simulink model "wlan_agc"  (Simulink 7.8)
settings: Solver=VariableStepDiscrete  SolverMode=SingleTasking  StartTime=0.0  StopTime=1e4  RelTol=1e-3
PostLoadFcn:
  | wlan_agc_init
InitFcn:
  | wlan_agc_init
StartFcn:
  | wlan_agc_init
undefined symbols (not defined in the file): gcbh, PHY_CONFIG_PKT_DET_CORR_THRESH, PHY_CONFIG_PKT_DET_ENERGY_THRESH, PHY_CONFIG_PKT_DET_MIN_DURR, xlBlockLoadCallback, xlGetNormalizedPeriod
libraries: xbsIndex_r4 x991, xbsEDKLib_r4 x1, simulink x1
(part 4 of 7)

== system wlan_agc/DCO Correction/DCO Corr1 ==
  IQ Valid : Inport
  I : Inport  Port=2
  Q : Inport  Port=3
  Accumulator : xbsIndex_r4/Accumulator  operation=Add  n_bits=17  overflow=Flag as error  scale=1  rst=on  infoeditControl=reset for floating point data type must be asserted for a minimum of 2 cycles  hasbypass=off  en=on  latency=0  dbl_ovrd=off  msb_inp=100  msb=100  lsb=-100  use_behavioral_HDL=on  implementation=Fabric  block_type=accum
      settings: block_version=VER_STRING_GOES_HERE
  Accumulator1 : xbsIndex_r4/Accumulator  operation=Add  n_bits=17  overflow=Flag as error  scale=1  rst=on  infoeditControl=reset for floating point data type must be asserted for a minimum of 2 cycles  hasbypass=off  en=on  latency=0  dbl_ovrd=off  msb_inp=100  msb=100  lsb=-100  use_behavioral_HDL=on  implementation=Fabric  block_type=accum
      settings: block_version=VER_STRING_GOES_HERE
  AddSub : xbsIndex_r4/AddSub  mode=Subtraction  use_carryin=off  use_carryout=off  en=off  latency=1  precision=User Defined  arith_type="Signed  (2's comp)"  n_bits=16  bin_pt=15  quantization=Truncate  overflow=Wrap  dbl_ovrd=off  use_behavioral_HDL=off  hw_selection=Fabric  pipelined=off  block_type=addsub
  AddSub1 : xbsIndex_r4/AddSub  mode=Subtraction  use_carryin=off  use_carryout=off  en=off  latency=1  precision=User Defined  arith_type="Signed  (2's comp)"  n_bits=16  bin_pt=15  quantization=Truncate  overflow=Wrap  dbl_ovrd=off  use_behavioral_HDL=off  hw_selection=Fabric  pipelined=off  block_type=addsub
  Constant : xbsIndex_r4/Constant  const=31  gui_display_data_type=Fixed-point  arith_type=Unsigned  n_bits=5  bin_pt=0  preci_type=Single  exp_width=8  frac_width=24  explicit_period=off  period=1  equ=P=C  opselect=C  inp2=PCIN>>17  opr=+  inp1=P  carry=CIN  dbl_ovrd=off  block_type=constant
  Counter : xbsIndex_r4/Counter  cnt_type=Free Running  cnt_to=Inf  operation=Up  start_count=0  cnt_by_val=1  arith_type=Unsigned  n_bits=5  bin_pt=0  load_pin=off  rst=on  en=on  explicit_period=off  period=1  dbl_ovrd=off  use_behavioral_HDL=off  implementation=Fabric  block_type=counter
  DCO Est : Scope  NumInputPorts=7
      settings: TimeRange=10000  YMin=-0.4~-0.4~0~0~-0.02~-0.4~-0.4  YMax=0.4~0.4~1~0.03~0.009999999999999999~0.4~0.4
  Delay : xbsIndex_r4/Delay  rst=off  infoeditControl=Selection of Reset will increase slice count due to use of real FFs and instead of SRLs  en=off  latency=1  dbl_ovrd=off  reg_retiming=off  block_type=delay
  Logical : xbsIndex_r4/Logical  logical_function=AND  inputs=2  en=off  latency=0  precision=Full  arith_type=Unsigned  n_bits=16  bin_pt=0  align_bp=on  dbl_ovrd=off  block_type=logical
  Logical1 : xbsIndex_r4/Logical  logical_function=OR  inputs=2  en=off  latency=0  precision=Full  arith_type=Unsigned  n_bits=16  bin_pt=0  align_bp=on  dbl_ovrd=off  block_type=logical
  Logical2 : xbsIndex_r4/Logical  logical_function=AND  inputs=2  en=off  latency=0  precision=Full  arith_type=Unsigned  n_bits=16  bin_pt=0  align_bp=on  dbl_ovrd=off  block_type=logical
  Relational : xbsIndex_r4/Relational  mode=a=b  en=off  latency=0  dbl_ovrd=off  block_type=relational
  S-R Latch : Subsystem
  Scale : xbsIndex_r4/Scale  scale_factor=-5  dbl_ovrd=off  block_type=scale
  Scale1 : xbsIndex_r4/Scale  scale_factor=-5  dbl_ovrd=off  block_type=scale
  done{1..7} (7 alike) : xbsIndex_r4/Gateway Out  inherit_from_input=off  hdl_port=off  timing_constraint=None  locs_specified=off  LOCs={}  UseAsDAC=off  DACChannel='1'  block_type=gatewayout
      settings: infoedit="Gateway out block.  Converts Xilinx fixed point inputs into ouputs of type Simulink integer, double, or fixed point.<P><P>Hardware notes:  In hardware these blocks become top level output ports or are discarded, depending on how they are configured."  xl_area=[0 0 0 0 1 0 0]  block_version=VER_STRING_GOES_HERE
  Valid : Outport
  " I" : Outport  Port=2
  " Q" : Outport  Port=3
  wires:
  done7/1 -> DCO Est/7
  done1/1 -> DCO Est/6
  done3/1 -> DCO Est/4
  done5/1 -> DCO Est/3
  done6/1 -> DCO Est/5
  done2/1 -> DCO Est/2
  done4/1 -> DCO Est/1
  Scale1/1 -> done6/1, AddSub1/2
  Scale/1 -> done3/1, AddSub/2
  Logical2/1 -> Logical1/2
  Relational/1 -> Logical2/2
  Delay/1 -> Valid/1
  AddSub1/1 -> done7/1, " Q"/1
  AddSub/1 -> done1/1, " I"/1
  Logical1/1 -> Counter/1, S-R Latch/2(R)
  [AGC_RESET] -> Logical1/1
  Accumulator1/1 -> Scale1/1
  Accumulator/1 -> Scale/1
  IQ Valid/1 -> Logical2/1, Logical/1, Delay/1
  S-R Latch/1(Q) -> Logical/2
  Counter/1 -> Relational/1
  Constant/1 -> Relational/2
  Logical/1 -> done5/1, Accumulator/3, Accumulator1/3, Counter/2
  [AGC_CTRL_Start_DCO] -> S-R Latch/1(S)
  [AGC_RESET] -> Accumulator/2, Accumulator1/2
  Q/1 -> done2/1, AddSub1/1, Accumulator1/1
  I/1 -> done4/1, AddSub/1, Accumulator/1

== system wlan_agc/DCO Correction/DCO Corr2 ==
  IQ Valid : Inport
  I : Inport  Port=2
  Q : Inport  Port=3
  Accumulator : xbsIndex_r4/Accumulator  operation=Add  n_bits=17  overflow=Flag as error  scale=1  rst=on  infoeditControl=reset for floating point data type must be asserted for a minimum of 2 cycles  hasbypass=off  en=on  latency=0  dbl_ovrd=off  msb_inp=100  msb=100  lsb=-100  use_behavioral_HDL=on  implementation=Fabric  block_type=accum
      settings: block_version=VER_STRING_GOES_HERE
  Accumulator1 : xbsIndex_r4/Accumulator  operation=Add  n_bits=17  overflow=Flag as error  scale=1  rst=on  infoeditControl=reset for floating point data type must be asserted for a minimum of 2 cycles  hasbypass=off  en=on  latency=0  dbl_ovrd=off  msb_inp=100  msb=100  lsb=-100  use_behavioral_HDL=on  implementation=Fabric  block_type=accum
      settings: block_version=VER_STRING_GOES_HERE
  AddSub : xbsIndex_r4/AddSub  mode=Subtraction  use_carryin=off  use_carryout=off  en=off  latency=1  precision=User Defined  arith_type="Signed  (2's comp)"  n_bits=16  bin_pt=15  quantization=Truncate  overflow=Wrap  dbl_ovrd=off  use_behavioral_HDL=off  hw_selection=Fabric  pipelined=off  block_type=addsub
  AddSub1 : xbsIndex_r4/AddSub  mode=Subtraction  use_carryin=off  use_carryout=off  en=off  latency=1  precision=User Defined  arith_type="Signed  (2's comp)"  n_bits=16  bin_pt=15  quantization=Truncate  overflow=Wrap  dbl_ovrd=off  use_behavioral_HDL=off  hw_selection=Fabric  pipelined=off  block_type=addsub
  Constant : xbsIndex_r4/Constant  const=31  gui_display_data_type=Fixed-point  arith_type=Unsigned  n_bits=5  bin_pt=0  preci_type=Single  exp_width=8  frac_width=24  explicit_period=off  period=1  equ=P=C  opselect=C  inp2=PCIN>>17  opr=+  inp1=P  carry=CIN  dbl_ovrd=off  block_type=constant
  Counter : xbsIndex_r4/Counter  cnt_type=Free Running  cnt_to=Inf  operation=Up  start_count=0  cnt_by_val=1  arith_type=Unsigned  n_bits=5  bin_pt=0  load_pin=off  rst=on  en=on  explicit_period=off  period=1  dbl_ovrd=off  use_behavioral_HDL=off  implementation=Fabric  block_type=counter
  DCO Est : Scope  NumInputPorts=7
      settings: TimeRange=10000  YMin=-0.4~-0.4~0~0~-0.02~-0.4~-0.4  YMax=0.4~0.4~1~0.03~0.009999999999999999~0.4~0.4
  Delay : xbsIndex_r4/Delay  rst=off  infoeditControl=Selection of Reset will increase slice count due to use of real FFs and instead of SRLs  en=off  latency=1  dbl_ovrd=off  reg_retiming=off  block_type=delay
  Logical : xbsIndex_r4/Logical  logical_function=AND  inputs=2  en=off  latency=0  precision=Full  arith_type=Unsigned  n_bits=16  bin_pt=0  align_bp=on  dbl_ovrd=off  block_type=logical
  Logical1 : xbsIndex_r4/Logical  logical_function=OR  inputs=2  en=off  latency=0  precision=Full  arith_type=Unsigned  n_bits=16  bin_pt=0  align_bp=on  dbl_ovrd=off  block_type=logical
  Logical2 : xbsIndex_r4/Logical  logical_function=AND  inputs=2  en=off  latency=0  precision=Full  arith_type=Unsigned  n_bits=16  bin_pt=0  align_bp=on  dbl_ovrd=off  block_type=logical
  Relational : xbsIndex_r4/Relational  mode=a=b  en=off  latency=0  dbl_ovrd=off  block_type=relational
  S-R Latch : Subsystem
  Scale : xbsIndex_r4/Scale  scale_factor=-5  dbl_ovrd=off  block_type=scale
  Scale1 : xbsIndex_r4/Scale  scale_factor=-5  dbl_ovrd=off  block_type=scale
  done{1..7} (7 alike) : xbsIndex_r4/Gateway Out  inherit_from_input=off  hdl_port=off  timing_constraint=None  locs_specified=off  LOCs={}  UseAsDAC=off  DACChannel='1'  block_type=gatewayout
      settings: infoedit="Gateway out block.  Converts Xilinx fixed point inputs into ouputs of type Simulink integer, double, or fixed point.<P><P>Hardware notes:  In hardware these blocks become top level output ports or are discarded, depending on how they are configured."  xl_area=[0 0 0 0 1 0 0]  block_version=VER_STRING_GOES_HERE
  Valid : Outport
  " I" : Outport  Port=2
  " Q" : Outport  Port=3
  wires:
  I/1 -> Accumulator/1, AddSub/1, done4/1
  Q/1 -> Accumulator1/1, AddSub1/1, done2/1
  [AGC_RESET] -> Accumulator1/2, Accumulator/2
  [AGC_CTRL_Start_DCO] -> S-R Latch/1(S)
  Logical/1 -> Counter/2, Accumulator1/3, Accumulator/3, done5/1
  Constant/1 -> Relational/2
  Counter/1 -> Relational/1
  S-R Latch/1(Q) -> Logical/2
  IQ Valid/1 -> Delay/1, Logical/1, Logical2/1
  Accumulator/1 -> Scale/1
  Accumulator1/1 -> Scale1/1
  [AGC_RESET] -> Logical1/1
  Logical1/1 -> S-R Latch/2(R), Counter/1
  AddSub/1 -> " I"/1, done1/1
  AddSub1/1 -> " Q"/1, done7/1
  Delay/1 -> Valid/1
  Relational/1 -> Logical2/2
  Logical2/1 -> Logical1/2
  Scale/1 -> AddSub/2, done3/1
  Scale1/1 -> AddSub1/2, done6/1
  done4/1 -> DCO Est/1
  done2/1 -> DCO Est/2
  done6/1 -> DCO Est/5
  done5/1 -> DCO Est/3
  done3/1 -> DCO Est/4
  done1/1 -> DCO Est/6
  done7/1 -> DCO Est/7

== system wlan_agc/DCO Correction/DCO Corr3 ==
  IQ Valid : Inport
  I : Inport  Port=2
  Q : Inport  Port=3
  Accumulator : xbsIndex_r4/Accumulator  operation=Add  n_bits=17  overflow=Flag as error  scale=1  rst=on  infoeditControl=reset for floating point data type must be asserted for a minimum of 2 cycles  hasbypass=off  en=on  latency=0  dbl_ovrd=off  msb_inp=100  msb=100  lsb=-100  use_behavioral_HDL=on  implementation=Fabric  block_type=accum
      settings: block_version=VER_STRING_GOES_HERE
  Accumulator1 : xbsIndex_r4/Accumulator  operation=Add  n_bits=17  overflow=Flag as error  scale=1  rst=on  infoeditControl=reset for floating point data type must be asserted for a minimum of 2 cycles  hasbypass=off  en=on  latency=0  dbl_ovrd=off  msb_inp=100  msb=100  lsb=-100  use_behavioral_HDL=on  implementation=Fabric  block_type=accum
      settings: block_version=VER_STRING_GOES_HERE
  AddSub : xbsIndex_r4/AddSub  mode=Subtraction  use_carryin=off  use_carryout=off  en=off  latency=1  precision=User Defined  arith_type="Signed  (2's comp)"  n_bits=16  bin_pt=15  quantization=Truncate  overflow=Wrap  dbl_ovrd=off  use_behavioral_HDL=off  hw_selection=Fabric  pipelined=off  block_type=addsub
  AddSub1 : xbsIndex_r4/AddSub  mode=Subtraction  use_carryin=off  use_carryout=off  en=off  latency=1  precision=User Defined  arith_type="Signed  (2's comp)"  n_bits=16  bin_pt=15  quantization=Truncate  overflow=Wrap  dbl_ovrd=off  use_behavioral_HDL=off  hw_selection=Fabric  pipelined=off  block_type=addsub
  Constant : xbsIndex_r4/Constant  const=31  gui_display_data_type=Fixed-point  arith_type=Unsigned  n_bits=5  bin_pt=0  preci_type=Single  exp_width=8  frac_width=24  explicit_period=off  period=1  equ=P=C  opselect=C  inp2=PCIN>>17  opr=+  inp1=P  carry=CIN  dbl_ovrd=off  block_type=constant
  Counter : xbsIndex_r4/Counter  cnt_type=Free Running  cnt_to=Inf  operation=Up  start_count=0  cnt_by_val=1  arith_type=Unsigned  n_bits=5  bin_pt=0  load_pin=off  rst=on  en=on  explicit_period=off  period=1  dbl_ovrd=off  use_behavioral_HDL=off  implementation=Fabric  block_type=counter
  DCO Est : Scope  NumInputPorts=7
      settings: TimeRange=10000  YMin=-0.4~-0.4~0~0~-0.02~-0.4~-0.4  YMax=0.4~0.4~1~0.03~0.009999999999999999~0.4~0.4
  Delay : xbsIndex_r4/Delay  rst=off  infoeditControl=Selection of Reset will increase slice count due to use of real FFs and instead of SRLs  en=off  latency=1  dbl_ovrd=off  reg_retiming=off  block_type=delay
  Logical : xbsIndex_r4/Logical  logical_function=AND  inputs=2  en=off  latency=0  precision=Full  arith_type=Unsigned  n_bits=16  bin_pt=0  align_bp=on  dbl_ovrd=off  block_type=logical
  Logical1 : xbsIndex_r4/Logical  logical_function=OR  inputs=2  en=off  latency=0  precision=Full  arith_type=Unsigned  n_bits=16  bin_pt=0  align_bp=on  dbl_ovrd=off  block_type=logical
  Logical2 : xbsIndex_r4/Logical  logical_function=AND  inputs=2  en=off  latency=0  precision=Full  arith_type=Unsigned  n_bits=16  bin_pt=0  align_bp=on  dbl_ovrd=off  block_type=logical
  Relational : xbsIndex_r4/Relational  mode=a=b  en=off  latency=0  dbl_ovrd=off  block_type=relational
  S-R Latch : Subsystem
  Scale : xbsIndex_r4/Scale  scale_factor=-5  dbl_ovrd=off  block_type=scale
  Scale1 : xbsIndex_r4/Scale  scale_factor=-5  dbl_ovrd=off  block_type=scale
  done{1..7} (7 alike) : xbsIndex_r4/Gateway Out  inherit_from_input=off  hdl_port=off  timing_constraint=None  locs_specified=off  LOCs={}  UseAsDAC=off  DACChannel='1'  block_type=gatewayout
      settings: infoedit="Gateway out block.  Converts Xilinx fixed point inputs into ouputs of type Simulink integer, double, or fixed point.<P><P>Hardware notes:  In hardware these blocks become top level output ports or are discarded, depending on how they are configured."  xl_area=[0 0 0 0 1 0 0]  block_version=VER_STRING_GOES_HERE
  Valid : Outport
  " I" : Outport  Port=2
  " Q" : Outport  Port=3
  wires:
  done7/1 -> DCO Est/7
  done1/1 -> DCO Est/6
  done3/1 -> DCO Est/4
  done5/1 -> DCO Est/3
  done6/1 -> DCO Est/5
  done2/1 -> DCO Est/2
  done4/1 -> DCO Est/1
  Scale1/1 -> done6/1, AddSub1/2
  Scale/1 -> done3/1, AddSub/2
  Logical2/1 -> Logical1/2
  Relational/1 -> Logical2/2
  Delay/1 -> Valid/1
  AddSub1/1 -> done7/1, " Q"/1
  AddSub/1 -> done1/1, " I"/1
  Logical1/1 -> Counter/1, S-R Latch/2(R)
  [AGC_RESET] -> Logical1/1
  Accumulator1/1 -> Scale1/1
  Accumulator/1 -> Scale/1
  IQ Valid/1 -> Logical2/1, Logical/1, Delay/1
  S-R Latch/1(Q) -> Logical/2
  Counter/1 -> Relational/1
  Constant/1 -> Relational/2
  Logical/1 -> done5/1, Accumulator/3, Accumulator1/3, Counter/2
  [AGC_CTRL_Start_DCO] -> S-R Latch/1(S)
  [AGC_RESET] -> Accumulator/2, Accumulator1/2
  Q/1 -> done2/1, AddSub1/1, Accumulator1/1
  I/1 -> done4/1, AddSub/1, Accumulator/1

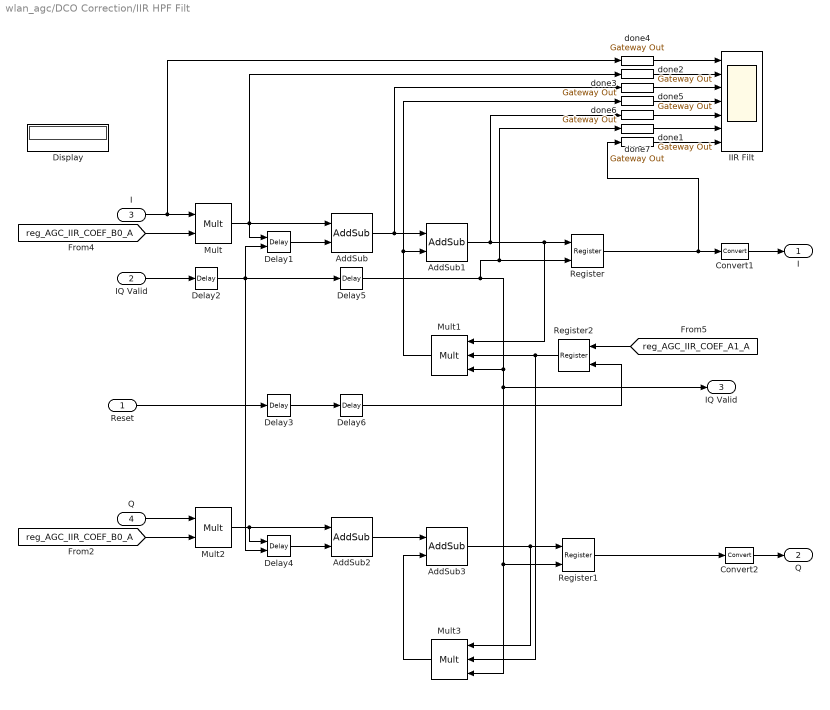
== system wlan_agc/DCO Correction/IIR HPF Filt ==
  Reset : Inport
  IQ Valid : Inport  Port=2
  I : Inport  Port=3
  Q : Inport  Port=4
  AddSub : xbsIndex_r4/AddSub  mode=Subtraction  use_carryin=off  use_carryout=off  en=off  latency=1  precision=Full  arith_type="Signed  (2's comp)"  n_bits=16  bin_pt=14  quantization=Truncate  overflow=Flag as error  dbl_ovrd=off  use_behavioral_HDL=off  hw_selection=Fabric  pipelined=off  block_type=addsub
  AddSub1 : xbsIndex_r4/AddSub  mode=Subtraction  use_carryin=off  use_carryout=off  en=off  latency=0  precision=Full  arith_type="Signed  (2's comp)"  n_bits=16  bin_pt=14  quantization=Truncate  overflow=Flag as error  dbl_ovrd=off  use_behavioral_HDL=off  hw_selection=Fabric  pipelined=off  block_type=addsub
  AddSub2 : xbsIndex_r4/AddSub  mode=Subtraction  use_carryin=off  use_carryout=off  en=off  latency=1  precision=Full  arith_type="Signed  (2's comp)"  n_bits=16  bin_pt=14  quantization=Truncate  overflow=Flag as error  dbl_ovrd=off  use_behavioral_HDL=off  hw_selection=Fabric  pipelined=off  block_type=addsub
  AddSub3 : xbsIndex_r4/AddSub  mode=Subtraction  use_carryin=off  use_carryout=off  en=off  latency=0  precision=Full  arith_type="Signed  (2's comp)"  n_bits=16  bin_pt=14  quantization=Truncate  overflow=Flag as error  dbl_ovrd=off  use_behavioral_HDL=off  hw_selection=Fabric  pipelined=off  block_type=addsub
  Convert1 : xbsIndex_r4/Convert  gui_display_data_type=Fixed-point  arith_type="Signed  (2's comp)"  n_bits=16  bin_pt=15  float_type=Single  exp_bits=8  fraction_bits=24  quantization=Truncate  overflow=Saturate  en=off  latency=0  dbl_ovrd=off  pipeline=off  block_type=convert
  Convert2 : xbsIndex_r4/Convert  gui_display_data_type=Fixed-point  arith_type="Signed  (2's comp)"  n_bits=16  bin_pt=15  float_type=Single  exp_bits=8  fraction_bits=24  quantization=Truncate  overflow=Saturate  en=off  latency=0  dbl_ovrd=off  pipeline=off  block_type=convert
  Delay1 : xbsIndex_r4/Delay  rst=off  infoeditControl=Selection of Reset will increase slice count due to use of real FFs and instead of SRLs  en=on  latency=1  dbl_ovrd=off  reg_retiming=off  block_type=delay
  Delay{2..3,5..6} (4 alike) : xbsIndex_r4/Delay  rst=off  infoeditControl=Selection of Reset will increase slice count due to use of real FFs and instead of SRLs  en=off  latency=1  dbl_ovrd=off  reg_retiming=off  block_type=delay
  Delay4 : xbsIndex_r4/Delay  rst=off  infoeditControl=Selection of Reset will increase slice count due to use of real FFs and instead of SRLs  en=on  latency=1  dbl_ovrd=off  reg_retiming=off  block_type=delay
  Display : Display
  IIR Filt : Scope  NumInputPorts=7
      settings: TimeRange=10000  YMin=-0.4~-0.4~-0.4~-1~-0.4~0~-0.4  YMax=0.4~0.4~0.4~1~0.4~1~0.4
  Mult : xbsIndex_r4/Mult  precision=User Defined  arith_type="Signed  (2's comp)"  n_bits=18  bin_pt=17  quantization=Truncate  overflow=Flag as error  en=off  latency=1  dbl_ovrd=off  use_behavioral_HDL=off  opt=Speed  use_embedded=on  optimum_pipeline=off  pipeline=on  use_rpm=on  placement_style=Triangular  block_type=mult
  Mult1 : xbsIndex_r4/Mult  precision=User Defined  arith_type="Signed  (2's comp)"  n_bits=18  bin_pt=16  quantization=Truncate  overflow=Flag as error  en=on  latency=1  dbl_ovrd=off  use_behavioral_HDL=off  opt=Speed  use_embedded=on  optimum_pipeline=off  pipeline=on  use_rpm=on  placement_style=Triangular  block_type=mult
  Mult2 : xbsIndex_r4/Mult  precision=User Defined  arith_type="Signed  (2's comp)"  n_bits=18  bin_pt=17  quantization=Truncate  overflow=Flag as error  en=off  latency=1  dbl_ovrd=off  use_behavioral_HDL=off  opt=Speed  use_embedded=on  optimum_pipeline=off  pipeline=on  use_rpm=on  placement_style=Triangular  block_type=mult
  Mult3 : xbsIndex_r4/Mult  precision=User Defined  arith_type="Signed  (2's comp)"  n_bits=18  bin_pt=16  quantization=Truncate  overflow=Flag as error  en=on  latency=1  dbl_ovrd=off  use_behavioral_HDL=off  opt=Speed  use_embedded=on  optimum_pipeline=off  pipeline=on  use_rpm=on  placement_style=Triangular  block_type=mult
  Register : xbsIndex_r4/Register  init=0  rst=off  en=on  dbl_ovrd=off  block_type=register
  Register1 : xbsIndex_r4/Register  init=0  rst=off  en=on  dbl_ovrd=off  block_type=register
  Register2 : xbsIndex_r4/Register  init=0  rst=on  en=off  dbl_ovrd=off  block_type=register
  done{1..7} (7 alike) : xbsIndex_r4/Gateway Out  inherit_from_input=off  hdl_port=off  timing_constraint=None  locs_specified=off  LOCs={}  UseAsDAC=off  DACChannel='1'  block_type=gatewayout
      settings: infoedit="Gateway out block.  Converts Xilinx fixed point inputs into ouputs of type Simulink integer, double, or fixed point.<P><P>Hardware notes:  In hardware these blocks become top level output ports or are discarded, depending on how they are configured."  xl_area=[0 0 0 0 1 0 0]  block_version=VER_STRING_GOES_HERE
  " I" : Outport
  " Q" : Outport  Port=2
  " IQ Valid" : Outport  Port=3
  wires:
  done2/1 -> IIR Filt/2
  done4/1 -> IIR Filt/1
  I/1 -> Mult/1, done4/1
  [reg_AGC_IIR_COEF_B0_A] -> Mult/2
  Mult/1 -> Delay1/1, AddSub/1, done2/1
  done1/1 -> IIR Filt/7
  done3/1 -> IIR Filt/3
  Delay1/1 -> AddSub/2
  AddSub/1 -> AddSub1/1, done3/1
  Mult1/1 -> AddSub1/2, done5/1
  done5/1 -> IIR Filt/4
  IQ Valid/1 -> Delay2/1
  Delay2/1 -> Delay1/2, Delay4/2, Delay5/1
  AddSub1/1 -> done6/1, Register/1, Mult1/1
  Register/1 -> done1/1, Convert1/1
  done6/1 -> IIR Filt/5
  done7/1 -> IIR Filt/6
  Q/1 -> Mult2/1
  [reg_AGC_IIR_COEF_B0_A] -> Mult2/2
  Mult2/1 -> Delay4/1, AddSub2/1
  Delay4/1 -> AddSub2/2
  AddSub2/1 -> AddSub3/1
  Mult3/1 -> AddSub3/2
  Convert1/1 -> " I"/1
  Convert2/1 -> " Q"/1
  Register2/1 -> Mult1/2, Mult3/2
  AddSub3/1 -> Register1/1, Mult3/1
  Register1/1 -> Convert2/1
  [reg_AGC_IIR_COEF_A1_A] -> Register2/1
  Reset/1 -> Delay3/1
  Delay3/1 -> Delay6/1
  Delay5/1 -> done7/1, Register/2, " IQ Valid"/1, Mult3/3, Register1/2, Mult1/3
  Delay6/1 -> Register2/2

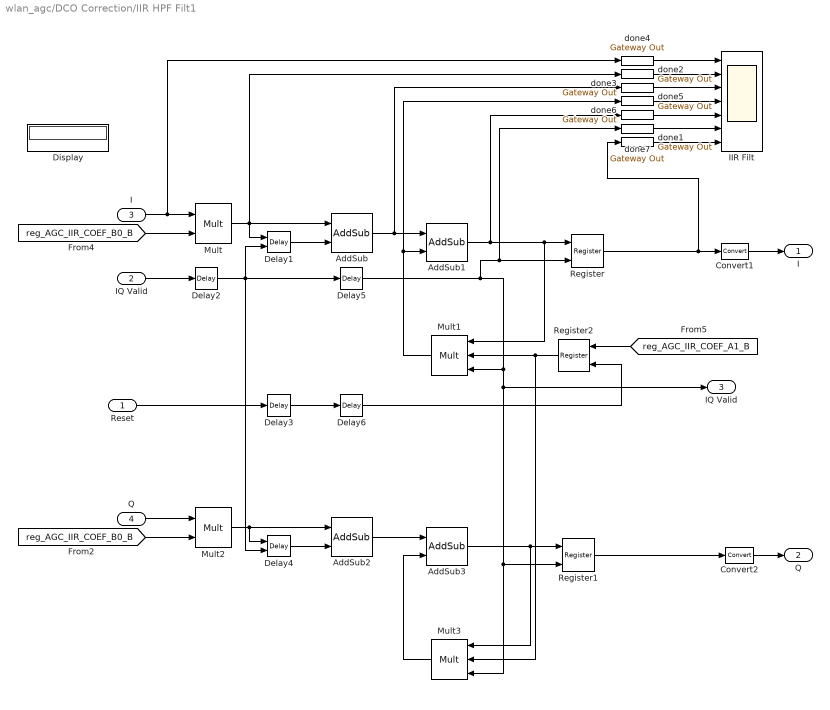
== system wlan_agc/DCO Correction/IIR HPF Filt1 ==
  Reset : Inport
  IQ Valid : Inport  Port=2
  I : Inport  Port=3
  Q : Inport  Port=4
  AddSub : xbsIndex_r4/AddSub  mode=Subtraction  use_carryin=off  use_carryout=off  en=off  latency=1  precision=Full  arith_type="Signed  (2's comp)"  n_bits=16  bin_pt=14  quantization=Truncate  overflow=Flag as error  dbl_ovrd=off  use_behavioral_HDL=off  hw_selection=Fabric  pipelined=off  block_type=addsub
  AddSub1 : xbsIndex_r4/AddSub  mode=Subtraction  use_carryin=off  use_carryout=off  en=off  latency=0  precision=Full  arith_type="Signed  (2's comp)"  n_bits=16  bin_pt=14  quantization=Truncate  overflow=Flag as error  dbl_ovrd=off  use_behavioral_HDL=off  hw_selection=Fabric  pipelined=off  block_type=addsub
  AddSub2 : xbsIndex_r4/AddSub  mode=Subtraction  use_carryin=off  use_carryout=off  en=off  latency=1  precision=Full  arith_type="Signed  (2's comp)"  n_bits=16  bin_pt=14  quantization=Truncate  overflow=Flag as error  dbl_ovrd=off  use_behavioral_HDL=off  hw_selection=Fabric  pipelined=off  block_type=addsub
  AddSub3 : xbsIndex_r4/AddSub  mode=Subtraction  use_carryin=off  use_carryout=off  en=off  latency=0  precision=Full  arith_type="Signed  (2's comp)"  n_bits=16  bin_pt=14  quantization=Truncate  overflow=Flag as error  dbl_ovrd=off  use_behavioral_HDL=off  hw_selection=Fabric  pipelined=off  block_type=addsub
  Convert1 : xbsIndex_r4/Convert  gui_display_data_type=Fixed-point  arith_type="Signed  (2's comp)"  n_bits=16  bin_pt=15  float_type=Single  exp_bits=8  fraction_bits=24  quantization=Truncate  overflow=Saturate  en=off  latency=0  dbl_ovrd=off  pipeline=off  block_type=convert
  Convert2 : xbsIndex_r4/Convert  gui_display_data_type=Fixed-point  arith_type="Signed  (2's comp)"  n_bits=16  bin_pt=15  float_type=Single  exp_bits=8  fraction_bits=24  quantization=Truncate  overflow=Saturate  en=off  latency=0  dbl_ovrd=off  pipeline=off  block_type=convert
  Delay1 : xbsIndex_r4/Delay  rst=off  infoeditControl=Selection of Reset will increase slice count due to use of real FFs and instead of SRLs  en=on  latency=1  dbl_ovrd=off  reg_retiming=off  block_type=delay
  Delay{2..3,5..6} (4 alike) : xbsIndex_r4/Delay  rst=off  infoeditControl=Selection of Reset will increase slice count due to use of real FFs and instead of SRLs  en=off  latency=1  dbl_ovrd=off  reg_retiming=off  block_type=delay
  Delay4 : xbsIndex_r4/Delay  rst=off  infoeditControl=Selection of Reset will increase slice count due to use of real FFs and instead of SRLs  en=on  latency=1  dbl_ovrd=off  reg_retiming=off  block_type=delay
  Display : Display
  IIR Filt : Scope  NumInputPorts=7
      settings: TimeRange=10000  YMin=-0.4~-0.4~-0.4~-1~-0.4~0~-0.4  YMax=0.4~0.4~0.4~1~0.4~1~0.4
  Mult : xbsIndex_r4/Mult  precision=User Defined  arith_type="Signed  (2's comp)"  n_bits=18  bin_pt=17  quantization=Truncate  overflow=Flag as error  en=off  latency=1  dbl_ovrd=off  use_behavioral_HDL=off  opt=Speed  use_embedded=on  optimum_pipeline=off  pipeline=on  use_rpm=on  placement_style=Triangular  block_type=mult
  Mult1 : xbsIndex_r4/Mult  precision=User Defined  arith_type="Signed  (2's comp)"  n_bits=18  bin_pt=16  quantization=Truncate  overflow=Flag as error  en=on  latency=1  dbl_ovrd=off  use_behavioral_HDL=off  opt=Speed  use_embedded=on  optimum_pipeline=off  pipeline=on  use_rpm=on  placement_style=Triangular  block_type=mult
  Mult2 : xbsIndex_r4/Mult  precision=User Defined  arith_type="Signed  (2's comp)"  n_bits=18  bin_pt=17  quantization=Truncate  overflow=Flag as error  en=off  latency=1  dbl_ovrd=off  use_behavioral_HDL=off  opt=Speed  use_embedded=on  optimum_pipeline=off  pipeline=on  use_rpm=on  placement_style=Triangular  block_type=mult
  Mult3 : xbsIndex_r4/Mult  precision=User Defined  arith_type="Signed  (2's comp)"  n_bits=18  bin_pt=16  quantization=Truncate  overflow=Flag as error  en=on  latency=1  dbl_ovrd=off  use_behavioral_HDL=off  opt=Speed  use_embedded=on  optimum_pipeline=off  pipeline=on  use_rpm=on  placement_style=Triangular  block_type=mult
  Register : xbsIndex_r4/Register  init=0  rst=off  en=on  dbl_ovrd=off  block_type=register
  Register1 : xbsIndex_r4/Register  init=0  rst=off  en=on  dbl_ovrd=off  block_type=register
  Register2 : xbsIndex_r4/Register  init=0  rst=on  en=off  dbl_ovrd=off  block_type=register
  done{1..7} (7 alike) : xbsIndex_r4/Gateway Out  inherit_from_input=off  hdl_port=off  timing_constraint=None  locs_specified=off  LOCs={}  UseAsDAC=off  DACChannel='1'  block_type=gatewayout
      settings: infoedit="Gateway out block.  Converts Xilinx fixed point inputs into ouputs of type Simulink integer, double, or fixed point.<P><P>Hardware notes:  In hardware these blocks become top level output ports or are discarded, depending on how they are configured."  xl_area=[0 0 0 0 1 0 0]  block_version=VER_STRING_GOES_HERE
  " I" : Outport
  " Q" : Outport  Port=2
  " IQ Valid" : Outport  Port=3
  wires:
  Delay6/1 -> Register2/2
  Delay5/1 -> Mult1/3, Register1/2, Mult3/3, " IQ Valid"/1, Register/2, done7/1
  Delay3/1 -> Delay6/1
  Reset/1 -> Delay3/1
  [reg_AGC_IIR_COEF_A1_B] -> Register2/1
  Register1/1 -> Convert2/1
  AddSub3/1 -> Mult3/1, Register1/1
  Register2/1 -> Mult3/2, Mult1/2
  Convert2/1 -> " Q"/1
  Convert1/1 -> " I"/1
  Mult3/1 -> AddSub3/2
  AddSub2/1 -> AddSub3/1
  Delay4/1 -> AddSub2/2
  Mult2/1 -> AddSub2/1, Delay4/1
  [reg_AGC_IIR_COEF_B0_B] -> Mult2/2
  Q/1 -> Mult2/1
  done7/1 -> IIR Filt/6
  done6/1 -> IIR Filt/5
  Register/1 -> Convert1/1, done1/1
  AddSub1/1 -> Mult1/1, Register/1, done6/1
  Delay2/1 -> Delay5/1, Delay4/2, Delay1/2
  IQ Valid/1 -> Delay2/1
  done5/1 -> IIR Filt/4
  Mult1/1 -> done5/1, AddSub1/2
  AddSub/1 -> done3/1, AddSub1/1
  Delay1/1 -> AddSub/2
  done3/1 -> IIR Filt/3
  done1/1 -> IIR Filt/7
  Mult/1 -> done2/1, AddSub/1, Delay1/1
  [reg_AGC_IIR_COEF_B0_B] -> Mult/2
  I/1 -> done4/1, Mult/1
  done4/1 -> IIR Filt/1
  done2/1 -> IIR Filt/2

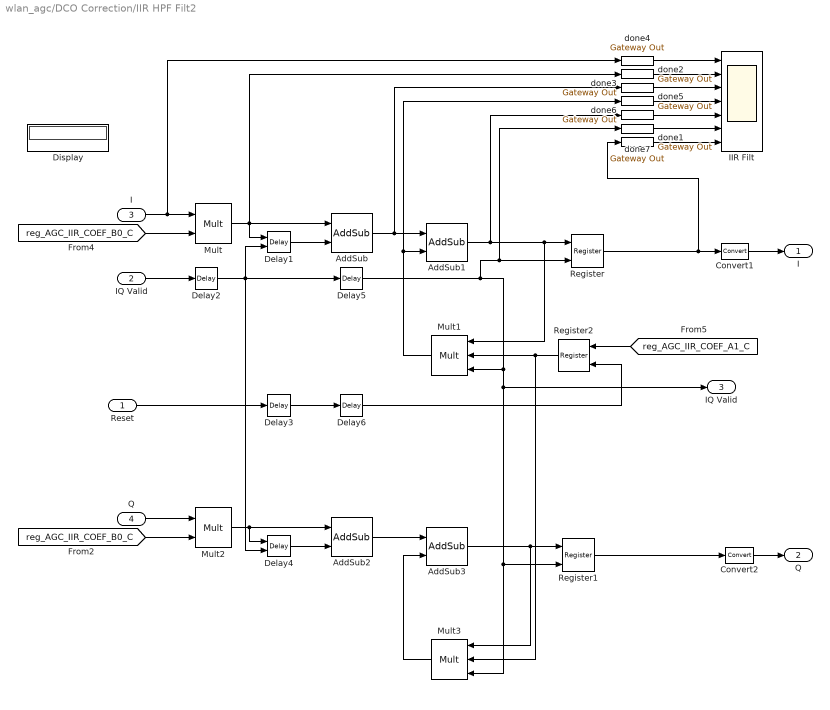
== system wlan_agc/DCO Correction/IIR HPF Filt2 ==
  Reset : Inport
  IQ Valid : Inport  Port=2
  I : Inport  Port=3
  Q : Inport  Port=4
  AddSub : xbsIndex_r4/AddSub  mode=Subtraction  use_carryin=off  use_carryout=off  en=off  latency=1  precision=Full  arith_type="Signed  (2's comp)"  n_bits=16  bin_pt=14  quantization=Truncate  overflow=Flag as error  dbl_ovrd=off  use_behavioral_HDL=off  hw_selection=Fabric  pipelined=off  block_type=addsub
  AddSub1 : xbsIndex_r4/AddSub  mode=Subtraction  use_carryin=off  use_carryout=off  en=off  latency=0  precision=Full  arith_type="Signed  (2's comp)"  n_bits=16  bin_pt=14  quantization=Truncate  overflow=Flag as error  dbl_ovrd=off  use_behavioral_HDL=off  hw_selection=Fabric  pipelined=off  block_type=addsub
  AddSub2 : xbsIndex_r4/AddSub  mode=Subtraction  use_carryin=off  use_carryout=off  en=off  latency=1  precision=Full  arith_type="Signed  (2's comp)"  n_bits=16  bin_pt=14  quantization=Truncate  overflow=Flag as error  dbl_ovrd=off  use_behavioral_HDL=off  hw_selection=Fabric  pipelined=off  block_type=addsub
  AddSub3 : xbsIndex_r4/AddSub  mode=Subtraction  use_carryin=off  use_carryout=off  en=off  latency=0  precision=Full  arith_type="Signed  (2's comp)"  n_bits=16  bin_pt=14  quantization=Truncate  overflow=Flag as error  dbl_ovrd=off  use_behavioral_HDL=off  hw_selection=Fabric  pipelined=off  block_type=addsub
  Convert1 : xbsIndex_r4/Convert  gui_display_data_type=Fixed-point  arith_type="Signed  (2's comp)"  n_bits=16  bin_pt=15  float_type=Single  exp_bits=8  fraction_bits=24  quantization=Truncate  overflow=Saturate  en=off  latency=0  dbl_ovrd=off  pipeline=off  block_type=convert
  Convert2 : xbsIndex_r4/Convert  gui_display_data_type=Fixed-point  arith_type="Signed  (2's comp)"  n_bits=16  bin_pt=15  float_type=Single  exp_bits=8  fraction_bits=24  quantization=Truncate  overflow=Saturate  en=off  latency=0  dbl_ovrd=off  pipeline=off  block_type=convert
  Delay1 : xbsIndex_r4/Delay  rst=off  infoeditControl=Selection of Reset will increase slice count due to use of real FFs and instead of SRLs  en=on  latency=1  dbl_ovrd=off  reg_retiming=off  block_type=delay
  Delay{2..3,5..6} (4 alike) : xbsIndex_r4/Delay  rst=off  infoeditControl=Selection of Reset will increase slice count due to use of real FFs and instead of SRLs  en=off  latency=1  dbl_ovrd=off  reg_retiming=off  block_type=delay
  Delay4 : xbsIndex_r4/Delay  rst=off  infoeditControl=Selection of Reset will increase slice count due to use of real FFs and instead of SRLs  en=on  latency=1  dbl_ovrd=off  reg_retiming=off  block_type=delay
  Display : Display
  IIR Filt : Scope  NumInputPorts=7
      settings: TimeRange=10000  YMin=-0.4~-0.4~-0.4~-1~-0.4~0~-0.4  YMax=0.4~0.4~0.4~1~0.4~1~0.4
  Mult : xbsIndex_r4/Mult  precision=User Defined  arith_type="Signed  (2's comp)"  n_bits=18  bin_pt=17  quantization=Truncate  overflow=Flag as error  en=off  latency=1  dbl_ovrd=off  use_behavioral_HDL=off  opt=Speed  use_embedded=on  optimum_pipeline=off  pipeline=on  use_rpm=on  placement_style=Triangular  block_type=mult
  Mult1 : xbsIndex_r4/Mult  precision=User Defined  arith_type="Signed  (2's comp)"  n_bits=18  bin_pt=16  quantization=Truncate  overflow=Flag as error  en=on  latency=1  dbl_ovrd=off  use_behavioral_HDL=off  opt=Speed  use_embedded=on  optimum_pipeline=off  pipeline=on  use_rpm=on  placement_style=Triangular  block_type=mult
  Mult2 : xbsIndex_r4/Mult  precision=User Defined  arith_type="Signed  (2's comp)"  n_bits=18  bin_pt=17  quantization=Truncate  overflow=Flag as error  en=off  latency=1  dbl_ovrd=off  use_behavioral_HDL=off  opt=Speed  use_embedded=on  optimum_pipeline=off  pipeline=on  use_rpm=on  placement_style=Triangular  block_type=mult
  Mult3 : xbsIndex_r4/Mult  precision=User Defined  arith_type="Signed  (2's comp)"  n_bits=18  bin_pt=16  quantization=Truncate  overflow=Flag as error  en=on  latency=1  dbl_ovrd=off  use_behavioral_HDL=off  opt=Speed  use_embedded=on  optimum_pipeline=off  pipeline=on  use_rpm=on  placement_style=Triangular  block_type=mult
  Register : xbsIndex_r4/Register  init=0  rst=off  en=on  dbl_ovrd=off  block_type=register
  Register1 : xbsIndex_r4/Register  init=0  rst=off  en=on  dbl_ovrd=off  block_type=register
  Register2 : xbsIndex_r4/Register  init=0  rst=on  en=off  dbl_ovrd=off  block_type=register
  done{1..7} (7 alike) : xbsIndex_r4/Gateway Out  inherit_from_input=off  hdl_port=off  timing_constraint=None  locs_specified=off  LOCs={}  UseAsDAC=off  DACChannel='1'  block_type=gatewayout
      settings: infoedit="Gateway out block.  Converts Xilinx fixed point inputs into ouputs of type Simulink integer, double, or fixed point.<P><P>Hardware notes:  In hardware these blocks become top level output ports or are discarded, depending on how they are configured."  xl_area=[0 0 0 0 1 0 0]  block_version=VER_STRING_GOES_HERE
  " I" : Outport
  " Q" : Outport  Port=2
  " IQ Valid" : Outport  Port=3
  wires:
  done2/1 -> IIR Filt/2
  done4/1 -> IIR Filt/1
  I/1 -> Mult/1, done4/1
  [reg_AGC_IIR_COEF_B0_C] -> Mult/2
  Mult/1 -> Delay1/1, AddSub/1, done2/1
  done1/1 -> IIR Filt/7
  done3/1 -> IIR Filt/3
  Delay1/1 -> AddSub/2
  AddSub/1 -> AddSub1/1, done3/1
  Mult1/1 -> AddSub1/2, done5/1
  done5/1 -> IIR Filt/4
  IQ Valid/1 -> Delay2/1
  Delay2/1 -> Delay1/2, Delay4/2, Delay5/1
  AddSub1/1 -> done6/1, Register/1, Mult1/1
  Register/1 -> done1/1, Convert1/1
  done6/1 -> IIR Filt/5
  done7/1 -> IIR Filt/6
  Q/1 -> Mult2/1
  [reg_AGC_IIR_COEF_B0_C] -> Mult2/2
  Mult2/1 -> Delay4/1, AddSub2/1
  Delay4/1 -> AddSub2/2
  AddSub2/1 -> AddSub3/1
  Mult3/1 -> AddSub3/2
  Convert1/1 -> " I"/1
  Convert2/1 -> " Q"/1
  Register2/1 -> Mult1/2, Mult3/2
  AddSub3/1 -> Register1/1, Mult3/1
  Register1/1 -> Convert2/1
  [reg_AGC_IIR_COEF_A1_C] -> Register2/1
  Reset/1 -> Delay3/1
  Delay3/1 -> Delay6/1
  Delay5/1 -> done7/1, Register/2, " IQ Valid"/1, Mult3/3, Register1/2, Mult1/3
  Delay6/1 -> Register2/2

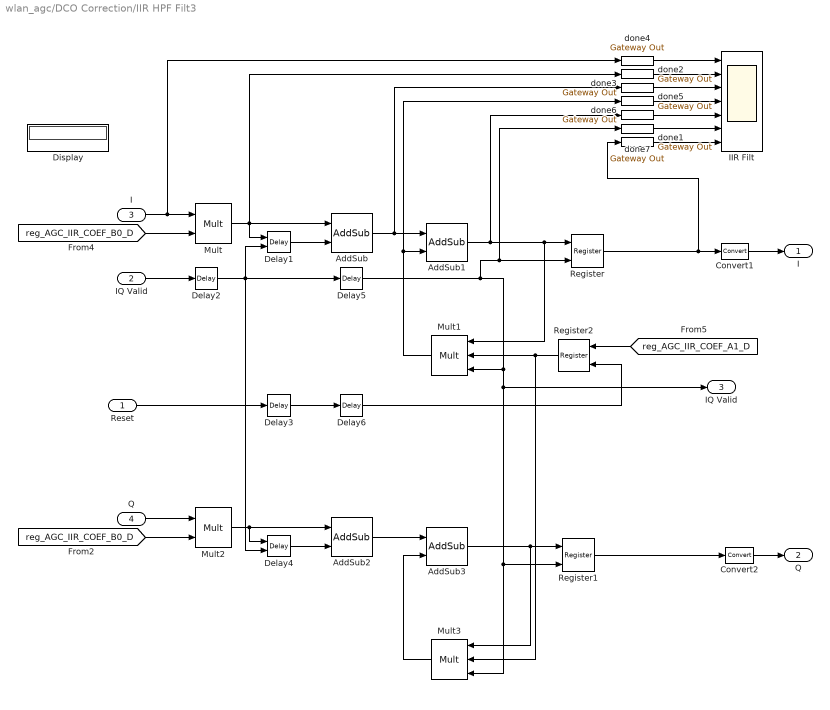
== system wlan_agc/DCO Correction/IIR HPF Filt3 ==
  Reset : Inport
  IQ Valid : Inport  Port=2
  I : Inport  Port=3
  Q : Inport  Port=4
  AddSub : xbsIndex_r4/AddSub  mode=Subtraction  use_carryin=off  use_carryout=off  en=off  latency=1  precision=Full  arith_type="Signed  (2's comp)"  n_bits=16  bin_pt=14  quantization=Truncate  overflow=Flag as error  dbl_ovrd=off  use_behavioral_HDL=off  hw_selection=Fabric  pipelined=off  block_type=addsub
  AddSub1 : xbsIndex_r4/AddSub  mode=Subtraction  use_carryin=off  use_carryout=off  en=off  latency=0  precision=Full  arith_type="Signed  (2's comp)"  n_bits=16  bin_pt=14  quantization=Truncate  overflow=Flag as error  dbl_ovrd=off  use_behavioral_HDL=off  hw_selection=Fabric  pipelined=off  block_type=addsub
  AddSub2 : xbsIndex_r4/AddSub  mode=Subtraction  use_carryin=off  use_carryout=off  en=off  latency=1  precision=Full  arith_type="Signed  (2's comp)"  n_bits=16  bin_pt=14  quantization=Truncate  overflow=Flag as error  dbl_ovrd=off  use_behavioral_HDL=off  hw_selection=Fabric  pipelined=off  block_type=addsub
  AddSub3 : xbsIndex_r4/AddSub  mode=Subtraction  use_carryin=off  use_carryout=off  en=off  latency=0  precision=Full  arith_type="Signed  (2's comp)"  n_bits=16  bin_pt=14  quantization=Truncate  overflow=Flag as error  dbl_ovrd=off  use_behavioral_HDL=off  hw_selection=Fabric  pipelined=off  block_type=addsub
  Convert1 : xbsIndex_r4/Convert  gui_display_data_type=Fixed-point  arith_type="Signed  (2's comp)"  n_bits=16  bin_pt=15  float_type=Single  exp_bits=8  fraction_bits=24  quantization=Truncate  overflow=Saturate  en=off  latency=0  dbl_ovrd=off  pipeline=off  block_type=convert
  Convert2 : xbsIndex_r4/Convert  gui_display_data_type=Fixed-point  arith_type="Signed  (2's comp)"  n_bits=16  bin_pt=15  float_type=Single  exp_bits=8  fraction_bits=24  quantization=Truncate  overflow=Saturate  en=off  latency=0  dbl_ovrd=off  pipeline=off  block_type=convert
  Delay1 : xbsIndex_r4/Delay  rst=off  infoeditControl=Selection of Reset will increase slice count due to use of real FFs and instead of SRLs  en=on  latency=1  dbl_ovrd=off  reg_retiming=off  block_type=delay
  Delay{2..3,5..6} (4 alike) : xbsIndex_r4/Delay  rst=off  infoeditControl=Selection of Reset will increase slice count due to use of real FFs and instead of SRLs  en=off  latency=1  dbl_ovrd=off  reg_retiming=off  block_type=delay
  Delay4 : xbsIndex_r4/Delay  rst=off  infoeditControl=Selection of Reset will increase slice count due to use of real FFs and instead of SRLs  en=on  latency=1  dbl_ovrd=off  reg_retiming=off  block_type=delay
  Display : Display
  IIR Filt : Scope  NumInputPorts=7
      settings: TimeRange=10000  YMin=-0.4~-0.4~-0.4~-1~-0.4~0~-0.4  YMax=0.4~0.4~0.4~1~0.4~1~0.4
  Mult : xbsIndex_r4/Mult  precision=User Defined  arith_type="Signed  (2's comp)"  n_bits=18  bin_pt=17  quantization=Truncate  overflow=Flag as error  en=off  latency=1  dbl_ovrd=off  use_behavioral_HDL=off  opt=Speed  use_embedded=on  optimum_pipeline=off  pipeline=on  use_rpm=on  placement_style=Triangular  block_type=mult
  Mult1 : xbsIndex_r4/Mult  precision=User Defined  arith_type="Signed  (2's comp)"  n_bits=18  bin_pt=16  quantization=Truncate  overflow=Flag as error  en=on  latency=1  dbl_ovrd=off  use_behavioral_HDL=off  opt=Speed  use_embedded=on  optimum_pipeline=off  pipeline=on  use_rpm=on  placement_style=Triangular  block_type=mult
  Mult2 : xbsIndex_r4/Mult  precision=User Defined  arith_type="Signed  (2's comp)"  n_bits=18  bin_pt=17  quantization=Truncate  overflow=Flag as error  en=off  latency=1  dbl_ovrd=off  use_behavioral_HDL=off  opt=Speed  use_embedded=on  optimum_pipeline=off  pipeline=on  use_rpm=on  placement_style=Triangular  block_type=mult
  Mult3 : xbsIndex_r4/Mult  precision=User Defined  arith_type="Signed  (2's comp)"  n_bits=18  bin_pt=16  quantization=Truncate  overflow=Flag as error  en=on  latency=1  dbl_ovrd=off  use_behavioral_HDL=off  opt=Speed  use_embedded=on  optimum_pipeline=off  pipeline=on  use_rpm=on  placement_style=Triangular  block_type=mult
  Register : xbsIndex_r4/Register  init=0  rst=off  en=on  dbl_ovrd=off  block_type=register
  Register1 : xbsIndex_r4/Register  init=0  rst=off  en=on  dbl_ovrd=off  block_type=register
  Register2 : xbsIndex_r4/Register  init=0  rst=on  en=off  dbl_ovrd=off  block_type=register
  done{1..7} (7 alike) : xbsIndex_r4/Gateway Out  inherit_from_input=off  hdl_port=off  timing_constraint=None  locs_specified=off  LOCs={}  UseAsDAC=off  DACChannel='1'  block_type=gatewayout
      settings: infoedit="Gateway out block.  Converts Xilinx fixed point inputs into ouputs of type Simulink integer, double, or fixed point.<P><P>Hardware notes:  In hardware these blocks become top level output ports or are discarded, depending on how they are configured."  xl_area=[0 0 0 0 1 0 0]  block_version=VER_STRING_GOES_HERE
  " I" : Outport
  " Q" : Outport  Port=2
  " IQ Valid" : Outport  Port=3
  wires:
  Delay6/1 -> Register2/2
  Delay5/1 -> Mult1/3, Register1/2, Mult3/3, " IQ Valid"/1, Register/2, done7/1
  Delay3/1 -> Delay6/1
  Reset/1 -> Delay3/1
  [reg_AGC_IIR_COEF_A1_D] -> Register2/1
  Register1/1 -> Convert2/1
  AddSub3/1 -> Mult3/1, Register1/1
  Register2/1 -> Mult3/2, Mult1/2
  Convert2/1 -> " Q"/1
  Convert1/1 -> " I"/1
  Mult3/1 -> AddSub3/2
  AddSub2/1 -> AddSub3/1
  Delay4/1 -> AddSub2/2
  Mult2/1 -> AddSub2/1, Delay4/1
  [reg_AGC_IIR_COEF_B0_D] -> Mult2/2
  Q/1 -> Mult2/1
  done7/1 -> IIR Filt/6
  done6/1 -> IIR Filt/5
  Register/1 -> Convert1/1, done1/1
  AddSub1/1 -> Mult1/1, Register/1, done6/1
  Delay2/1 -> Delay5/1, Delay4/2, Delay1/2
  IQ Valid/1 -> Delay2/1
  done5/1 -> IIR Filt/4
  Mult1/1 -> done5/1, AddSub1/2
  AddSub/1 -> done3/1, AddSub1/1
  Delay1/1 -> AddSub/2
  done3/1 -> IIR Filt/3
  done1/1 -> IIR Filt/7
  Mult/1 -> done2/1, AddSub/1, Delay1/1
  [reg_AGC_IIR_COEF_B0_D] -> Mult/2
  I/1 -> done4/1, Mult/1
  done4/1 -> IIR Filt/1
  done2/1 -> IIR Filt/2

== system wlan_agc/DCO Correction/S-R Latch ==
  S : Inport
  R : Inport  Port=2
  Constant1 : xbsIndex_r4/Constant  const=1  gui_display_data_type=Boolean  arith_type=Boolean  n_bits=1  bin_pt=0  preci_type=Single  exp_width=8  frac_width=24  explicit_period=off  period=1  equ=P=C  opselect=C  inp2=PCIN>>17  opr=+  inp1=P  carry=CIN  dbl_ovrd=off  block_type=constant
      settings: block_version=VER_STRING_GOES_HERE
  Register2 : xbsIndex_r4/Register  init=0  rst=on  en=on  dbl_ovrd=off  block_type=register
      settings: xl_area=[1 1 0 0 0 0 0]  block_version=VER_STRING_GOES_HERE
  Q : Outport
  wires:
  Constant1/1 -> Register2/1
  R/1 -> Register2/2
  Register2/1 -> Q/1
  S/1 -> Register2/3

== system wlan_agc/Gain Calc A/BB gain ==
  G_RF_dB : Inport
  P_IN_RSSI : Inport  Port=2
  IQ_dBv : Inport  Port=3
  AddSub : xbsIndex_r4/AddSub  mode=Subtraction  use_carryin=off  use_carryout=off  en=off  latency=1  precision=User Defined  arith_type="Signed  (2's comp)"  n_bits=8  bin_pt=0  quantization=Truncate  overflow=Wrap  dbl_ovrd=off  use_behavioral_HDL=off  hw_selection=Fabric  pipelined=off  block_type=addsub
  AddSub1 : xbsIndex_r4/AddSub  mode=Subtraction  use_carryin=off  use_carryout=off  en=off  latency=1  precision=User Defined  arith_type="Signed  (2's comp)"  n_bits=8  bin_pt=0  quantization=Truncate  overflow=Wrap  dbl_ovrd=off  use_behavioral_HDL=off  hw_selection=Fabric  pipelined=off  block_type=addsub
  AddSub2 : xbsIndex_r4/AddSub  mode=Subtraction  use_carryin=off  use_carryout=off  en=off  latency=0  precision=User Defined  arith_type="Signed  (2's comp)"  n_bits=8  bin_pt=0  quantization=Truncate  overflow=Wrap  dbl_ovrd=off  use_behavioral_HDL=off  hw_selection=Fabric  pipelined=off  block_type=addsub
  AddSub3 : xbsIndex_r4/AddSub  mode=Addition  use_carryin=off  use_carryout=off  en=off  latency=1  precision=User Defined  arith_type="Signed  (2's comp)"  n_bits=8  bin_pt=0  quantization=Truncate  overflow=Wrap  dbl_ovrd=off  use_behavioral_HDL=off  hw_selection=Fabric  pipelined=off  block_type=addsub
  AddSub4 : xbsIndex_r4/AddSub  mode=Subtraction  use_carryin=off  use_carryout=off  en=off  latency=0  precision=User Defined  arith_type="Signed  (2's comp)"  n_bits=8  bin_pt=0  quantization=Truncate  overflow=Wrap  dbl_ovrd=off  use_behavioral_HDL=off  hw_selection=Fabric  pipelined=off  block_type=addsub
  Convert1 : xbsIndex_r4/Convert  gui_display_data_type=Fixed-point  arith_type=Unsigned  n_bits=5  bin_pt=0  float_type=Single  exp_bits=8  fraction_bits=24  quantization=Truncate  overflow=Saturate  en=off  latency=0  dbl_ovrd=off  pipeline=off  block_type=convert
  Convert2 : xbsIndex_r4/Convert  gui_display_data_type=Fixed-point  arith_type=Unsigned  n_bits=5  bin_pt=0  float_type=Single  exp_bits=8  fraction_bits=24  quantization=Truncate  overflow=Saturate  en=off  latency=0  dbl_ovrd=off  pipeline=off  block_type=convert
  Mux : xbsIndex_r4/Mux  inputs=3  en=off  latency=0  precision=Full  arith_type=Unsigned  n_bits=16  bin_pt=14  quantization=Truncate  overflow=Wrap  dbl_ovrd=off  block_type=mux
  Shift : xbsIndex_r4/Shift  shift_dir=Right  shift_bits=1  en=off  latency=0  precision=Full  arith_type="Signed  (2's comp)"  n_bits=16  bin_pt=14  quantization=Truncate  overflow=Wrap  dbl_ovrd=off  block_type=shift
  Shift1 : xbsIndex_r4/Shift  shift_dir=Right  shift_bits=1  en=off  latency=0  precision=Full  arith_type="Signed  (2's comp)"  n_bits=16  bin_pt=14  quantization=Truncate  overflow=Wrap  dbl_ovrd=off  block_type=shift
  G_BB : Outport
  wires:
  [reg_AGC_INIT_G_BB] -> Mux/2
  [reg_AGC_TARGET_PWR] -> AddSub/1, AddSub2/1
  AddSub/1 -> AddSub1/1
  AddSub1/1 -> Shift/1, AddSub3/2
  Shift/1 -> Convert1/1
  AddSub2/1 -> AddSub3/1
  AddSub3/1 -> Shift1/1
  Shift1/1 -> Convert2/1
  Convert1/1 -> Mux/3
  Convert2/1 -> Mux/4
  G_RF_dB/1 -> AddSub1/2
  Mux/1 -> G_BB/1
  P_IN_RSSI/1 -> AddSub/2
  AddSub4/1 -> AddSub2/2
  [AGC_CTRL_G_BB_SEL] -> Mux/1
  IQ_dBv/1 -> AddSub4/1
  [reg_AGC_V_DB_ADJ] -> AddSub4/2

== system wlan_agc/Gain Calc A/Capture & Convert ==
  note: Shift slope-adjusted value by gain-dependent
      | offset (top-center plot on pg 16 of MAX2829 ds)
  G_RF : Inport
  RSSI : Inport  Port=2
  AddSub : xbsIndex_r4/AddSub  mode=Subtraction  use_carryin=off  use_carryout=off  en=off  latency=1  precision=User Defined  arith_type="Signed  (2's comp)"  n_bits=8  bin_pt=0  quantization=Truncate  overflow=Flag as error  dbl_ovrd=off  use_behavioral_HDL=off  hw_selection=Fabric  pipelined=off  block_type=addsub
  Constant : xbsIndex_r4/Constant  const=1/15  gui_display_data_type=Fixed-point  arith_type=Unsigned  n_bits=12  bin_pt=12  preci_type=Single  exp_width=8  frac_width=24  explicit_period=off  period=1  equ=P=C  opselect=C  inp2=PCIN>>17  opr=+  inp1=P  carry=CIN  dbl_ovrd=off  block_type=constant
  Constant1 : xbsIndex_r4/Constant  const=100  gui_display_data_type=Fixed-point  arith_type=Unsigned  n_bits=7  bin_pt=0  preci_type=Single  exp_width=8  frac_width=24  explicit_period=off  period=1  equ=P=C  opselect=C  inp2=PCIN>>17  opr=+  inp1=P  carry=CIN  dbl_ovrd=off  block_type=constant
  Constant2 : xbsIndex_r4/Constant  const=85  gui_display_data_type=Fixed-point  arith_type=Unsigned  n_bits=7  bin_pt=0  preci_type=Single  exp_width=8  frac_width=24  explicit_period=off  period=1  equ=P=C  opselect=C  inp2=PCIN>>17  opr=+  inp1=P  carry=CIN  dbl_ovrd=off  block_type=constant
  Constant3 : xbsIndex_r4/Constant  const=70  gui_display_data_type=Fixed-point  arith_type=Unsigned  n_bits=7  bin_pt=0  preci_type=Single  exp_width=8  frac_width=24  explicit_period=off  period=1  equ=P=C  opselect=C  inp2=PCIN>>17  opr=+  inp1=P  carry=CIN  dbl_ovrd=off  block_type=constant
  Display : Display
  Display1 : Display
  Display2 : Display
  Mult : xbsIndex_r4/Mult  precision=User Defined  arith_type=Unsigned  n_bits=11  bin_pt=4  quantization=Truncate  overflow=Wrap  en=off  latency=1  dbl_ovrd=off  use_behavioral_HDL=off  opt=Speed  use_embedded=on  optimum_pipeline=off  pipeline=on  use_rpm=on  placement_style=Triangular  block_type=mult
  Mux1 : xbsIndex_r4/Mux  inputs=4  en=off  latency=0  precision=Full  arith_type=Unsigned  n_bits=16  bin_pt=14  quantization=Truncate  overflow=Wrap  dbl_ovrd=off  block_type=mux
  RSSI Calc : Scope  NumInputPorts=7
      settings: TimeRange=10000  YMin=-1~-1~0~0~0~-40~-1  YMax=1~1~0.8~0.2~80~0~1  SaveName=ScopeData7
  Register : xbsIndex_r4/Register  init=3  rst=on  en=on  dbl_ovrd=off  block_type=register
  done{1..8} (8 alike) : xbsIndex_r4/Gateway Out  inherit_from_input=off  hdl_port=off  timing_constraint=None  locs_specified=off  LOCs={}  UseAsDAC=off  DACChannel='1'  block_type=gatewayout
      settings: infoedit="Gateway out block.  Converts Xilinx fixed point inputs into ouputs of type Simulink integer, double, or fixed point.<P><P>Hardware notes:  In hardware these blocks become top level output ports or are discarded, depending on how they are configured."  xl_area=[0 0 0 0 1 0 0]  block_version=VER_STRING_GOES_HERE
  Rx Pwr (dBm) : Outport
  wires:
  [AGC_CTRL_Capture_RSSI] -> Register/3, done5/1
  [AGC_RESET] -> Register/2
  RSSI/1 -> Register/1, done7/1
  Register/1 -> Mult/1, done1/1, done3/1
  Constant/1 -> Mult/2
  Mult/1 -> AddSub/1, done4/1
  Mux1/1 -> AddSub/2, done6/1
  AddSub/1 -> Rx Pwr (dBm)/1, done2/1, done8/1
  [reg_AGC_RSSI_CALIB_G1] -> Mux1/2, Mux1/3
  [reg_AGC_RSSI_CALIB_G2] -> Mux1/4
  [reg_AGC_RSSI_CALIB_G3] -> Mux1/5
  G_RF/1 -> Mux1/1
  done4/1 -> Display/1
  done1/1 -> Display1/1
  done2/1 -> Display2/1
  done7/1 -> RSSI Calc/1
  done5/1 -> RSSI Calc/2
  done3/1 -> RSSI Calc/3
  done6/1 -> RSSI Calc/4
  done8/1 -> RSSI Calc/5

== system wlan_agc/Gain Calc A/IQ Mag ==
  I : Inport
  Q : Inport  Port=2
  Valid : Inport  Port=3
  AddSub : xbsIndex_r4/AddSub  mode=Addition  use_carryin=off  use_carryout=off  en=off  latency=0  precision=User Defined  arith_type=Unsigned  n_bits=20  bin_pt=19  quantization=Truncate  overflow=Flag as error  dbl_ovrd=off  use_behavioral_HDL=off  hw_selection=Fabric  pipelined=off  block_type=addsub
  Delay : xbsIndex_r4/Delay  rst=off  infoeditControl=Selection of Reset will increase slice count due to use of real FFs and instead of SRLs  en=off  latency=1  dbl_ovrd=off  reg_retiming=off  block_type=delay
  Mult : xbsIndex_r4/Mult  precision=User Defined  arith_type=Unsigned  n_bits=20  bin_pt=20  quantization=Truncate  overflow=Saturate  en=off  latency=1  dbl_ovrd=off  use_behavioral_HDL=off  opt=Speed  use_embedded=on  optimum_pipeline=off  pipeline=on  use_rpm=on  placement_style=Triangular  block_type=mult
  Mult1 : xbsIndex_r4/Mult  precision=User Defined  arith_type=Unsigned  n_bits=20  bin_pt=20  quantization=Truncate  overflow=Saturate  en=off  latency=1  dbl_ovrd=off  use_behavioral_HDL=off  opt=Speed  use_embedded=on  optimum_pipeline=off  pipeline=on  use_rpm=on  placement_style=Triangular  block_type=mult
  ROM : xbsIndex_r4/ROM  depth=2^11  initVector=5*log10(linspace(2^-11, 2, 2048))  distributed_mem=Block RAM  rst=off  init_reg=0  en=off  latency=1  gui_display_data_type=Fixed-point  arith_type="Signed  (2's comp)"  n_bits=14  bin_pt=8  preci_type=Single  exp_width=8  frac_width=24  dbl_ovrd=off  optimize=Area  use_rpm=on  block_type=sprom
  Register : xbsIndex_r4/Register  init=0  rst=on  en=on  dbl_ovrd=off  block_type=register
  Reinterpret : xbsIndex_r4/Reinterpret  force_arith_type=off  arith_type=Unsigned  force_bin_pt=on  bin_pt=0  block_type=reinterpret
  Running Sum : Subsystem
  V_DB : Scope  NumInputPorts=7
      settings: TimeRange=10000  YMin=-0.75~-0.75~0~0~0~-17.5~-1  YMax=0.75~0.75~0.35~0.125~125~0~1  SaveName=ScopeData4
  done{1..7} (7 alike) : xbsIndex_r4/Gateway Out  inherit_from_input=off  hdl_port=off  timing_constraint=None  locs_specified=off  LOCs={}  UseAsDAC=off  DACChannel='1'  block_type=gatewayout
      settings: infoedit="Gateway out block.  Converts Xilinx fixed point inputs into ouputs of type Simulink integer, double, or fixed point.<P><P>Hardware notes:  In hardware these blocks become top level output ports or are discarded, depending on how they are configured."  xl_area=[0 0 0 0 1 0 0]  block_version=VER_STRING_GOES_HERE
  IQ_dBv : Outport
  wires:
  Delay/1 -> Running Sum/1(En)
  I/1 -> Mult/1, Mult/2, done4/1
  Valid/1 -> Delay/1
  Running Sum/1(Sum) -> Reinterpret/1, done3/1
  Q/1 -> Mult1/2, Mult1/1, done2/1
  Mult/1 -> AddSub/1
  Mult1/1 -> AddSub/2
  AddSub/1 -> Running Sum/2(D), done1/1
  ROM/1 -> Register/1, done6/1
  [AGC_CTRL_Capture_V_DB] -> Register/3, done7/1
  [AGC_DONE_G_BB] -> Register/2
  Register/1 -> IQ_dBv/1
  Reinterpret/1 -> ROM/1, done5/1
  done4/1 -> V_DB/1
  done2/1 -> V_DB/2
  done1/1 -> V_DB/3
  done3/1 -> V_DB/4
  done5/1 -> V_DB/5
  done6/1 -> V_DB/6
  done7/1 -> V_DB/7
